simulink model "blockmodel_16a"  (R2017b)
settings: Solver=VariableStepAuto  StartTime=0.0  StopTime=10  MaxStep=0.001  RelTol=1e-3
PreLoadFcn:
  | tic
values from neighbouring files (symbols this model uses):
  a = 1    [init.m]
  a_m = -4    [init.m]
  b = 3    [init.m]
  b_m = 4    [init.m]
  theta_f = [0.01 -1 1 0.5]    [init.m]
  x_m_0 = 0    [init.m]
  x_p_0 = 0    [init.m]
CloseFcn:
  | toc
settings Model: Creator=q3  LastModifiedBy=q3
settings OptimizationCC: LifeSpan=inf
settings DebuggingCC: SFExecutionAtInitializationDiag=none
settings CodeAppCC: StateflowObjectComments=on

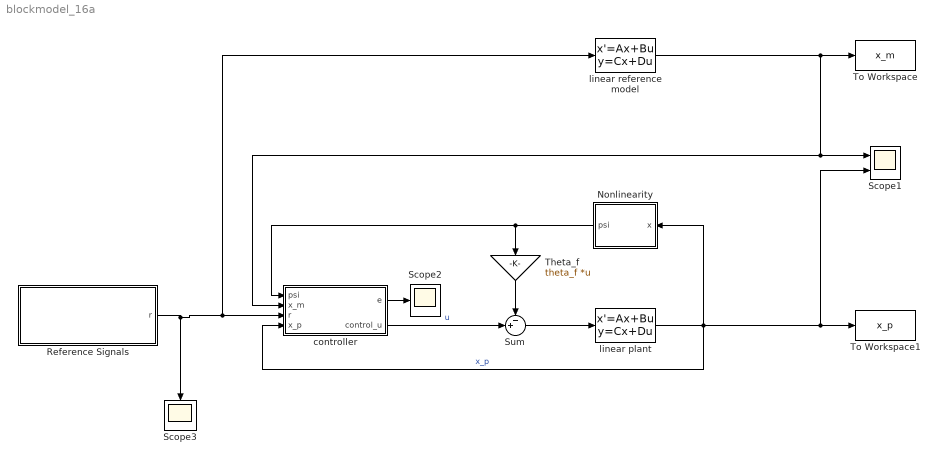
== system blockmodel_16a ==
  "Nonlinearity " : MATLAB Function  TreatAsAtomicUnit=on
  Reference Signals : Subsystem
  Scope1 : Scope  NumInputPorts=2
  Scope2 : Scope
  Scope3 : Scope
  Sum : Sum  Inputs=-+|
  Theta_f : Gain  Gain=theta_f  Multiplication=Matrix(K*u) (u vector)
  To Workspace : ToWorkspace  VariableName=x_m  SampleTime=-1
  To Workspace1 : ToWorkspace  VariableName=x_p  SampleTime=-1
  controller : Subsystem
  linear plant : StateSpace  A=a  B=b  D=0  InitialCondition=x_p_0
  linear reference model : StateSpace  A=a_m  B=b_m  D=0  InitialCondition=x_m_0
  wires:
  controller/1(e) -> Scope2/1
  Reference Signals/1(r) -> linear reference model/1, controller/3(r), Scope3/1
  controller/2(control_u) -> Sum/2  "u"
  "Nonlinearity "/1(psi) -> controller/1(psi), Theta_f/1
  linear reference model/1 -> Scope1/1, controller/2(x_m), To Workspace/1
  Theta_f/1 -> Sum/1
  Sum/1 -> linear plant/1
  linear plant/1 -> controller/4(x_p), Scope1/2, To Workspace1/1, "Nonlinearity "/1(x)  "x_p"

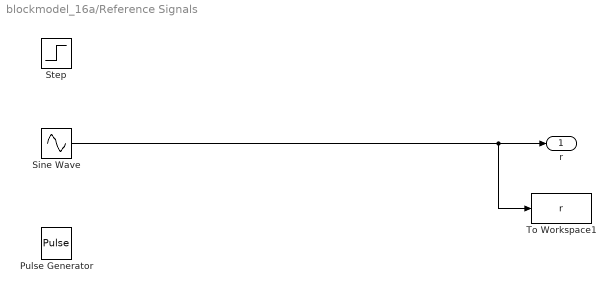
== system blockmodel_16a/Reference Signals ==
  Pulse Generator : DiscretePulseGenerator  PulseType=Time based  Amplitude=4  PulseWidth=50
  Sine Wave : Sin  Amplitude=4  Frequency=4  SampleTime=0
  Step : Step  After=4  SampleTime=0
  To Workspace1 : ToWorkspace  VariableName=r  SampleTime=-1
  r : Outport
  wires:
  Sine Wave/1 -> To Workspace1/1, r/1

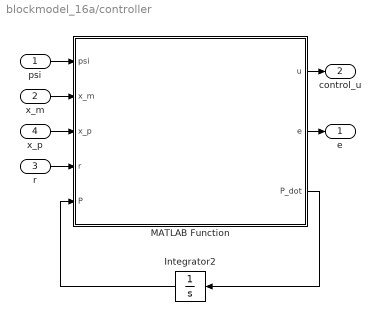
== system blockmodel_16a/controller ==
  psi : Inport
  x_m : Inport  Port=2
  r : Inport  Port=3
  x_p : Inport  Port=4
  Integrator2 : Integrator  InitialCondition=[0 0]
  MATLAB Function : MATLAB Function  TreatAsAtomicUnit=on
  e : Outport
  control_u : Outport  Port=2
  wires:
  x_p/1 -> MATLAB Function/3(x_p)
  MATLAB Function/1(u) -> control_u/1
  r/1 -> MATLAB Function/4(r)
  x_m/1 -> MATLAB Function/2(x_m)
  MATLAB Function/3(P_dot) -> Integrator2/1
  Integrator2/1 -> MATLAB Function/5(P)
  psi/1 -> MATLAB Function/1(psi)
  MATLAB Function/2(e) -> e/1

== matlab function blockmodel_16a/Nonlinearity  ==
  data: x input; psi output
function psi = fcn(x)

% Basisfunctions
psi = [x^3 exp(-10*(x+0.5)^2) exp(-10*(x-0.5)^2) sin(2*x)]';

== matlab function blockmodel_16a/controller/MATLAB Function ==
  data: psi input; u output; e output; x_m input; P_dot output; x_p input; r input; P input
function [u,e,P_dot] = fcn(psi,x_m,x_p,r,P)
theta = P(1);
k = P(2);
% adaptive gain
gamma = 2;

% error
e = x_p - x_m;

% adaptive law
theta_dot = -gamma*e*x_p;
k_dot = -gamma*e*r; 

P_dot = [theta_dot k_dot];

% control law
u = theta*x_p + k*r;
